simulink model "PMSM_self_test"  (R2021b)
settings: Solver=ode15s  StartTime=0.0  StopTime=1  RelTol=1e-3
values from neighbouring files (symbols this model uses):
  b = 0    [PMSM_self_code.m]
  J = 1.0000e-04    (= 0.0001)    [PMSM_self_code.m]
  Ld = 0.0057    [PMSM_self_code.m]
  Lq = 0.0125    [PMSM_self_code.m]
  P = 4    [PMSM_self_code.m]
  PM = 0.1230    (= 0.123)    [PMSM_self_code.m]
  r = 1.2000    (= 1.2)    [PMSM_self_code.m]
  Vp_p_amp = 220*sqrt(2)    [PMSM_self_code.m]
  w = 2*pi*f    (= 376.991118431)    [PMSM_self_code.m]
libraries: fl_lib x5, nesl_utility x4, ee_lib x3, spsabctodq0Lib x1, spsdq0toabcLib x1
settings Model: Creator=DELL  LastModifiedBy=DELL

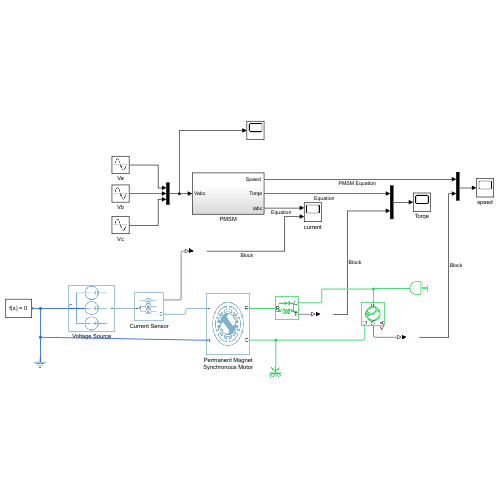
[thumbnail: Simulink's stored preview of the top-level diagram]
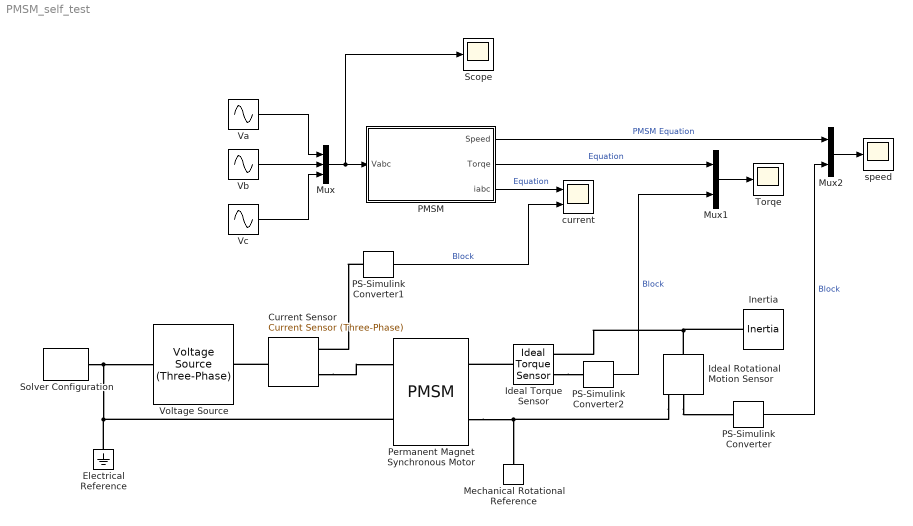
== system PMSM_self_test ==
  Current Sensor : ee_lib/Sensors & Transducers/Current Sensor (Three-Phase)
  Electrical Reference : fl_lib/Electrical/Electrical Elements/Electrical Reference
  Ideal Rotational Motion Sensor : fl_lib/Mechanical/Mechanical Sensors/Ideal Rotational Motion Sensor  wrap_angle=simscape.enum.onoff.off  offset=0 deg
  Ideal Torque Sensor : fl_lib/Mechanical/Mechanical Sensors/Ideal Torque Sensor
      settings: SourceProductName=Foundation Library
  Inertia : fl_lib/Mechanical/Rotational Elements/Inertia  inertia="0.0001  kg*m^2"  num_ports=foundation.enum.numPorts2.one  w_specify=off  w_priority=High  w=0 rad/s  w_nominal_specify=off  w_nominal_unit=rad/s  w_nominal_value=1  t_specify=off  t_priority=None  t=0 N*m  t_nominal_specify=off  t_nominal_unit=N*m  t_nominal_value=1
  Mechanical Rotational Reference : fl_lib/Mechanical/Rotational Elements/Mechanical Rotational Reference
  Mux : Mux  Inputs=3
  Mux1 : Mux  Inputs=2
  Mux2 : Mux  Inputs=2
  PMSM : Subsystem
  PS-Simulink Converter : nesl_utility/PS-Simulink Converter  PhysicalDomain=network_engine_domain  SubClassName=ps_output  LeftPortType=input  RightPortType=output  PseudoPeriodic=off  Frequencies=[]  Unit=rad/s  AffineConversion=off
  PS-Simulink Converter1 : nesl_utility/PS-Simulink Converter  PhysicalDomain=network_engine_domain  SubClassName=ps_output  LeftPortType=input  RightPortType=output  PseudoPeriodic=off  Frequencies=[]  Unit=A  AffineConversion=off
  PS-Simulink Converter2 : nesl_utility/PS-Simulink Converter  PhysicalDomain=network_engine_domain  SubClassName=ps_output  LeftPortType=input  RightPortType=output  PseudoPeriodic=off  Frequencies=[]  Unit=N*m  AffineConversion=off
  Permanent Magnet Synchronous Motor : ee_lib/Electromechanical/Permanent Magnet/PMSM  port_option=ee.enum.threePhasePort.composite  winding_type=ee.enum.statorconnection.wye  machine_param=ee.enum.pmsm.parameterization.constant  nPolePairs=P/2  pmflux_param=1  pm_flux_linkage=PM Wb  torque_constant=0.18 N*m/A  back_emf_constant=0.18 V/(rad/s)  stator_param=1  Ld=Ld H  Lq=Lq H  idVec=[-200, 0, 200] A  iqVec=[-200, 0, 200] A  LdMatrix=0.0002 * ones(3, 3) H  LqMatrix=0.0002 * ones(3, 3) H  PmMatrix=0.1 * ones(3, 3) Wb  ktMatrix=0.18 * ones(3, 3) N*m/A  keMatrix=0.18 * ones(3, 3) V*s/rad  L0=0 H  Ls=0.0002 H  Lm=-0.00002 H  Ms=0.00002 H  Rs=r Ohm  zero_sequence=ee.enum.park.zerosequence.include  axes_param=2  loss_param=ee.enum.ironloss.none  losses_oc=[0, 0, 0] W  losses_sc=[0, 0, 0] W  f_losses=60 Hz  Isc_losses=95 A  J=0 kg*m^2  lam=0 N*m*s/rad  i_d_specify=off  i_d_priority=None  i_d=0 A  i_d_nominal_specify=off  i_d_nominal_unit=A  i_d_nominal_value=1  i_q_specify=off  i_q_priority=None  i_q=0 A  i_q_nominal_specify=off  i_q_nominal_unit=A  i_q_nominal_value=1  torque_specify=off  torque_priority=None  torque=0 N*m  torque_nominal_specify=off  torque_nominal_unit=N*m  torque_nominal_value=1  angular_velocity_specify=on  angular_velocity_priority=None  angular_velocity=0 rpm  angular_velocity_nominal_specify=off  angular_velocity_nominal_unit=rpm  angular_velocity_nominal_value=1  angular_position_specify=on  angular_position_priority=High  angular_position=0 deg  angular_position_nominal_specify=off  angular_position_nominal_unit=deg  angular_position_nominal_value=1  alpha=3.93e-3 1/K  alpha_flux=-0.001 1/K  Tmeas=298.15 K  stator_thermal_mass=100 J/K  rotor_thermal_mass=200 J/K  Rm_percent_rotor=90  Rd_percent_rotor=30  temperatureA_specify=off  temperatureA_priority=High  temperatureA=25 degC  temperatureA_nominal_specify=off  temperatureA_nominal_unit=degC  temperatureA_nominal_value=1  temperatureB_specify=off  temperatureB_priority=High  temperatureB=25 degC  temperatureB_nominal_specify=off  temperatureB_nominal_unit=degC  temperatureB_nominal_value=1  temperatureC_specify=off  temperatureC_priority=High  temperatureC=25 degC  temperatureC_nominal_specify=off  temperatureC_nominal_unit=degC  temperatureC_nominal_value=1  temperatureR_specify=off  temperatureR_priority=High  temperatureR=25 degC  temperatureR_nominal_specify=off  temperatureR_nominal_unit=degC  temperatureR_nominal_value=1
      settings: InternalSimscapePortConfiguration="{\"Bottom\":[],\"Left\":[{\"id\":\"N\",\"label\":\"~\",\"type\":\"foundation.electrical.three_phase\"},{\"id\":\"n\",\"label\":\"n\",\"type\":\"foundation.electrical.electrical\"}],\"Right\":[{\"id\":\"R\",\"label\":\"R\",\"type\":\"foundation.mechanical.rotational.rotational\"},{\"id\":\"C\",\"label\":\"C\",\"type\":\"foundation.mechanical.rotational.rotational\"}],\"Top\":[]}"
  Scope : Scope
  Solver Configuration : nesl_utility/Solver Configuration  PhysicalDomain=network_engine_domain  SubClassName=solver  LeftPortType=input  RightPortType=generic  Tones=[]  Harmonics=[]  SimulateNoise=off  Profile=off  UseLocalSampling=off  EnableSwitchedLinearOptims=on  FrequencyDomain=off  UseCCode=off  RelTol=0.001  AbsTol=1e-06  MinStep=1e-09  ToWorkspace=off  RevertToSquareIcSolve=off  NumHomotopyIterations=100  PhasorMode=off  PhasorModeNumHarmonics=1  DoDC=off  ResidualTolerance=1e-09  UseLocalSolver=off  LocalSolverChoice=NE_BACKWARD_EULER_ADVANCER  LocalSolverSampleTime=0.001  DoFixedCost=off  MaxNonlinIter=3  MaxModeIter=2  ComputeImpulses=off  ImpulseIterations=2  LinearAlgebra=Sparse  EquationFormulation=NE_TIME_EF  DelaysMemoryBudget=1024  AutomaticFiltering=on  FilteringTimeConstant=0.001  PartitionStorageMethod=AS_NEEDED  PartitionMemoryBudget=1024  PartitionMethod=FAST
  "Torqe " : Scope
  Va : Sin  Amplitude=Vp_p_amp  Frequency=w  SampleTime=0
  Vb : Sin  Amplitude=Vp_p_amp  Frequency=w  Phase=-2*pi/3  SampleTime=0
  Vc : Sin  Amplitude=Vp_p_amp  Frequency=w  Phase=2*pi/3  SampleTime=0
  Voltage Source : ee_lib/Sources/Voltage Source (Three-Phase)  vline_rms=380 V  shift=0 deg  freq=60 Hz  impedance_option=0  SShortCircuit=1e6 V*A  XR=15  R=0.01 Ohm  L=3.97e-4 H  harmonic_option=0  harmonic_orders=[5, 7, 11, 13]  harmonic_ratios=[.1, .1, .1, .1]  G_parasitic=0 1/Ohm  I_specify=off  I_priority=None  I=[ 0 0 0 ] A  I_nominal_specify=off  I_nominal_unit=A  I_nominal_value=1
      settings: SourceProductBaseCode=PS
  current : Scope  NumInputPorts=2
  speed : Scope
  wires:
  Mux/1 -> Scope/1, PMSM/1(Vabc)
  PS-Simulink Converter/1 -> Mux2/2  "Block"
  PMSM/3(iabc) -> current/1  "Equation"
  Vc/1 -> Mux/3
  Mux1/1 -> "Torqe "/1
  PMSM/2(Torqe) -> Mux1/1  "Equation"
  PS-Simulink Converter1/1 -> current/2  "Block"
  PMSM/1("Speed ") -> Mux2/1  "PMSM Equation"
  PS-Simulink Converter2/1 -> Mux1/2  "Block"
  Mux2/1 -> speed/1
  Vb/1 -> Mux/2
  Va/1 -> Mux/1
  connections:
  Ideal Rotational Motion Sensor/RConn1 -- Permanent Magnet Synchronous Motor/RConn2 -- Mechanical Rotational Reference/LConn1
  Solver Configuration/RConn1 -- Voltage Source/LConn1 -- Electrical Reference/LConn1 -- Permanent Magnet Synchronous Motor/LConn2
  Ideal Torque Sensor/RConn1 -- Inertia/LConn1 -- Ideal Rotational Motion Sensor/LConn1
  Current Sensor/RConn2 -- Permanent Magnet Synchronous Motor/LConn1
  Ideal Rotational Motion Sensor/RConn2 -- PS-Simulink Converter/LConn1
  PS-Simulink Converter1/LConn1 -- Current Sensor/RConn1
  Current Sensor/LConn1 -- Voltage Source/RConn1
  Ideal Torque Sensor/LConn1 -- Permanent Magnet Synchronous Motor/RConn1
  Ideal Torque Sensor/RConn2 -- PS-Simulink Converter2/LConn1

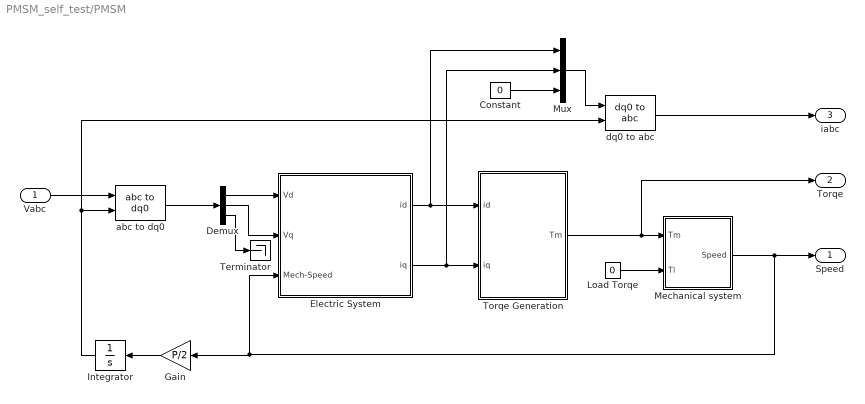
== system PMSM_self_test/PMSM ==
  Vabc : Inport
  Constant : Constant  Value=0
  Demux : Demux  Outputs=3
  "Electric System " : Subsystem
  Gain : Gain  Gain=P/2
  Integrator : Integrator
  Load Torqe : Constant  Value=0
  Mechanical system : Subsystem
  Mux : Mux  Inputs=3
  Terminator : Terminator
  Torqe Generation : Subsystem
  abc to dq0 : spsabctodq0Lib/abc to dq0  Alignment=Aligned with phase A axis
  dq0 to abc : spsdq0toabcLib/dq0 to abc  Alignment=90 degrees behind phase A axis
  "Speed " : Outport  VectorParamsAs1DForOutWhenUnconnected=off
  Torqe : Outport  Port=2  VectorParamsAs1DForOutWhenUnconnected=off
  iabc : Outport  Port=3  VectorParamsAs1DForOutWhenUnconnected=off
  wires:
  Load Torqe/1 -> Mechanical system/2(Tl)
  Demux/1 -> "Electric System "/1(Vd)
  Torqe Generation/1(Tm) -> Torqe/1, Mechanical system/1(Tm)
  Demux/2 -> "Electric System "/2("Vq ")
  Mechanical system/1(Speed) -> "Speed "/1, "Electric System "/3("Mech-Speed "), Gain/1
  "Electric System "/1("id ") -> Torqe Generation/1(id), Mux/1
  Vabc/1 -> abc to dq0/1
  "Electric System "/2(iq) -> Torqe Generation/2("iq "), Mux/2
  Gain/1 -> Integrator/1
  Integrator/1 -> dq0 to abc/2, abc to dq0/2
  dq0 to abc/1 -> iabc/1
  abc to dq0/1 -> Demux/1
  Demux/3 -> Terminator/1
  Constant/1 -> Mux/3
  Mux/1 -> dq0 to abc/1

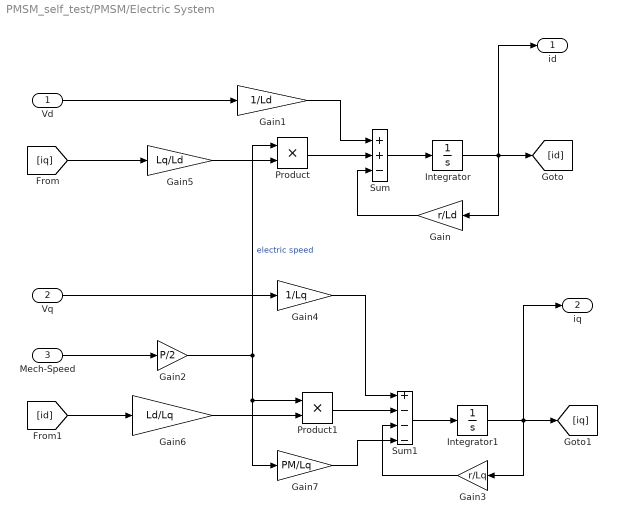
== system PMSM_self_test/PMSM/Electric System  ==
  Vd : Inport
  "Vq " : Inport  Port=2
  "Mech-Speed " : Inport  Port=3
  Gain : Gain  Gain=r/Ld
  Gain1 : Gain  Gain=1/Ld
  Gain2 : Gain  Gain=P/2
  Gain3 : Gain  Gain=r/Lq
  Gain4 : Gain  Gain=1/Lq
  Gain5 : Gain  Gain=Lq/Ld
  Gain6 : Gain  Gain=Ld/Lq
  Gain7 : Gain  Gain=PM/Lq
  Integrator : Integrator
  Integrator1 : Integrator
  Product : Product
  Product1 : Product
  Sum : Sum  Inputs=++-
  Sum1 : Sum  Inputs=+---
  "id " : Outport  VectorParamsAs1DForOutWhenUnconnected=off
  iq : Outport  Port=2  VectorParamsAs1DForOutWhenUnconnected=off
  wires:
  Integrator/1 -> "id "/1, [id], Gain/1
  Gain1/1 -> Sum/1
  Sum/1 -> Integrator/1
  Vd/1 -> Gain1/1
  Gain/1 -> Sum/3
  Product/1 -> Sum/2
  Gain3/1 -> Sum1/3
  Gain4/1 -> Sum1/1
  Product1/1 -> Sum1/2
  "Vq "/1 -> Gain4/1
  Sum1/1 -> Integrator1/1
  Integrator1/1 -> iq/1, [iq], Gain3/1
  "Mech-Speed "/1 -> Gain2/1
  Gain2/1 -> Gain7/1, Product1/1, Product/1  "electric speed"
  [iq] -> Gain5/1
  Gain5/1 -> Product/2
  [id] -> Gain6/1
  Gain6/1 -> Product1/2
  Gain7/1 -> Sum1/4

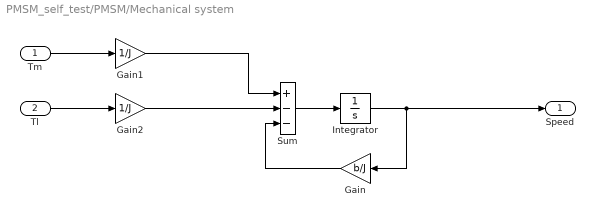
== system PMSM_self_test/PMSM/Mechanical system ==
  Tm : Inport
  Tl : Inport  Port=2
  Gain : Gain  Gain=b/J
  Gain1 : Gain  Gain=1/J
  Gain2 : Gain  Gain=1/J
  Integrator : Integrator
  Sum : Sum  Inputs=+--
  Speed : Outport  VectorParamsAs1DForOutWhenUnconnected=off
  wires:
  Integrator/1 -> Speed/1, Gain/1
  Gain1/1 -> Sum/1
  Gain2/1 -> Sum/2
  Sum/1 -> Integrator/1
  Gain/1 -> Sum/3
  Tm/1 -> Gain1/1
  Tl/1 -> Gain2/1

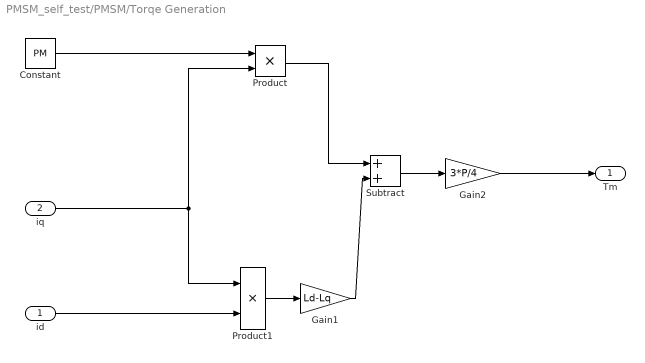
== system PMSM_self_test/PMSM/Torqe Generation ==
  id : Inport
  "iq " : Inport  Port=2
  Constant : Constant  Value=PM
  Gain1 : Gain  Gain=Ld-Lq
  Gain2 : Gain  Gain=3*P/4
  Product : Product
  Product1 : Product
  Subtract : Sum
  Tm : Outport  VectorParamsAs1DForOutWhenUnconnected=off
  wires:
  id/1 -> Product1/2
  Constant/1 -> Product/1
  "iq "/1 -> Product1/1, Product/2
  Product/1 -> Subtract/1
  Subtract/1 -> Gain2/1
  Gain2/1 -> Tm/1
  Product1/1 -> Gain1/1
  Gain1/1 -> Subtract/2
